simulink model "Kalman_filter_mod"  (R2020a)
settings: Solver=ode1  StartTime=0.0  StopTime=10.0  FixedStep=.05  RelTol=1e-3
values from neighbouring files (symbols this model uses):
  Aol = sys_d.A    [Kalman_filter.m]
  Bol = sys_d.B    [Kalman_filter.m]
  Col = sys_d.C    [Kalman_filter.m]
  L = 3.23    [Kalman_filter_Params1.m]    (also in UT.m = size(X,2); myMeasurementFcn.m; myStateTransitionFcn.m)
libraries: simulink x2
settings Model: Creator=NIKHIL  LastModifiedBy=NIKHIL

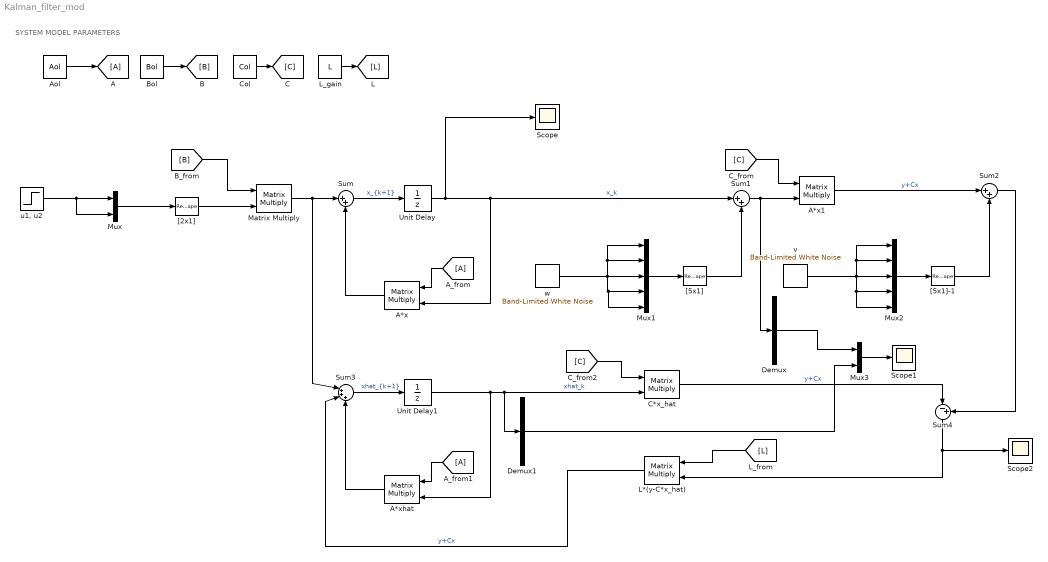
== system Kalman_filter_mod ==
  note: SYSTEM MODEL PARAMETERS
  A*x : Product  Multiplication=Matrix(*)
  A*x1 : Product  Multiplication=Matrix(*)
  A*xhat : Product  Multiplication=Matrix(*)
  Aol : Constant  Value=Aol
  Bol : Constant  Value=Bol
  C*x_hat : Product  Multiplication=Matrix(*)
  Col : Constant  Value=Col
  Demux : Demux  Outputs=5
  Demux1 : Demux  Outputs=5
  L*(y-C*x_hat) : Product  Multiplication=Matrix(*)
  L_gain : Constant  Value=L
  Matrix Multiply : Product  Multiplication=Matrix(*)
  Mux : Mux  Inputs=2
  Mux1 : Mux  Inputs=5
  Mux2 : Mux  Inputs=5
  Mux3 : Mux  Inputs=2
  Scope : Scope
  Scope1 : Scope
  Scope2 : Scope
  Sum : Sum  Inputs=|++
  Sum1 : Sum  Inputs=|++
  Sum2 : Sum  Inputs=|++
  Sum3 : Sum  Inputs=|+++
  Sum4 : Sum  Inputs=|-+
  Unit Delay : UnitDelay  SampleTime=-1  HasFrameUpgradeWarning=on
  Unit Delay1 : UnitDelay  SampleTime=-1  HasFrameUpgradeWarning=on
  "[2x1]" : Reshape  OutputDimensionality=Customize  OutputDimensions=[2,1]
  "[5x1]" : Reshape  OutputDimensionality=Customize  OutputDimensions=[5,1]
  "[5x1]-1" : Reshape  OutputDimensionality=Customize  OutputDimensions=[5,1]
  "u1, u2" : Step  SampleTime=0
  v : simulink/Sources/Band-Limited White Noise  Cov=[0.1]  Ts=0.05  seed=[23341]
  w : simulink/Sources/Band-Limited White Noise  Cov=[0.1]  Ts=0.05  seed=[23341]
  wires:
  Aol/1 -> [A]
  Bol/1 -> [B]
  Col/1 -> [C]
  L_gain/1 -> [L]
  "u1, u2"/1 -> Mux/2, Mux/1
  Mux/1 -> "[2x1]"/1
  "[2x1]"/1 -> Matrix Multiply/2
  [B] -> Matrix Multiply/1
  Matrix Multiply/1 -> Sum3/1, Sum/1
  Sum/1 -> Unit Delay/1  "x_{k+1}"
  Unit Delay/1 -> Scope/1, Sum1/1, A*x/2  "x_k"
  [A] -> A*x/1
  A*x/1 -> Sum/2
  w/1 -> Mux1/1, Mux1/2, Mux1/5, Mux1/4, Mux1/3
  Mux1/1 -> "[5x1]"/1
  "[5x1]"/1 -> Sum1/2
  Sum1/1 -> Demux/1, A*x1/2
  [C] -> A*x1/1
  "[5x1]-1"/1 -> Sum2/2
  Mux2/1 -> "[5x1]-1"/1
  v/1 -> Mux2/3, Mux2/4, Mux2/5, Mux2/2, Mux2/1
  A*x1/1 -> Sum2/1  "y+Cx"
  [A] -> A*xhat/1
  Unit Delay1/1 -> A*xhat/2, Demux1/1, C*x_hat/2  "xhat_k"
  Sum3/1 -> Unit Delay1/1  "xhat_{k+1}"
  A*xhat/1 -> Sum3/3
  [C] -> C*x_hat/1
  C*x_hat/1 -> Sum4/1  "y+Cx"
  Sum2/1 -> Sum4/2
  [L] -> L*(y-C*x_hat)/1
  Sum4/1 -> Scope2/1, L*(y-C*x_hat)/2
  L*(y-C*x_hat)/1 -> Sum3/2  "y+Cx"
  Demux/3 -> Mux3/1
  Demux1/3 -> Mux3/2
  Mux3/1 -> Scope1/1
